simulink model "sltestCustomSourceSinkExample"  (R2016a)
settings: Solver=FixedStepDiscrete  SolverMode=SingleTasking  StartTime=0.0  StopTime=10  FixedStep=0.01  RelTol=1e-5  AbsTol=1e-6
model workspace (MAT data in the model file):
  PressEst = [0.806253176324 0.553142316929 0.37151500209 0.277667903103 0.220198954207 0.181288665766 0.153200000489 0.115431020872 0.0913067476324 0.0746519188607 0.0625231108324 0.0533383634277 ... (306 elements, 18x17)]
  PressVect = [0.05 0.1 0.15 0.2 0.25 0.3 0.35 0.4 0.45 0.5 0.55 0.6 0.65 0.7 0.75 0.8 0.85 0.9 0.95]
  PumpCon = [-0.0556348 -0.0022828 0.0256932 0.0435188 0.0562692 0.0661194857143 0.0741572 0.08697 0.0972452 0.106070342857 0.1139892 0.121303866667 ... (342 elements, 18x19)]
  RampRateKiX = [100 200 300 400 500 600]
  RampRateKiY = [0 0.2 0.4 0.6 0.8 1]
  RampRateKiZ = [0.012  0.024  0.036  0.048  0.06  0.072; 0.024  0.048  0.072  0.096  0.12  0.144; 0.036  0.072  0.108  0.144  0.18  0.216; 0.048  0.096  0.144  0.192  0.24  0.288; 0.06  0.12  0.18  0.24  0.3  0.36; 0.072  0.144  0.216  0.288  0.36  0.432]
  SpeedEst = [471.837839721 550.80940091 777.559313277 1080.9243499 1418.36795322 1769.7468768 2125.37309264 2480.20345067 2831.37796793 3177.14006959 3516.32917143 4064.90417867 ... (323 elements, 17x19)]
  SpeedVect = [50 75 100 125 150 175 200 250 300 350 400 450 500 600 700 800 900 1000]
  ThrotEst = [0 0 0 0 0 0 0 0 0 0 0 0 ... (342 elements, 18x19)]
  ThrotVect = [0 3 6 9 12 15 18 21 24 27 30 35 46 57 68 79 90]
  hys = 25
  max_ego = 1.2
  max_press = 0.95
  max_speed = 628
  max_throt = 90
  min_press = 0.05
  min_speed = 50
  min_throt = 3
  st_range = 0.0001
  zero_thresh = 250
Description:
  | This is a model of a fuel control system where Stateflow(R) is used to handle the fault management of the system.
  | The system contains four separate sensors: a throttle sensor, a speed sensor, an oxygen sensor, and a pressure sensor.
  | Each of these sensors is represented by a parallel state in Stateflow.  Each parallel state contains two substates, a
  | normal state and a failed state (the exception being the oxygen sensor, which also contains a warmup state).
  | 
  | If any of the sensor readings is outside an acceptable range, then a fault is registered in Stateflow, and the
  | substate of the corresponding subsystem transitions to the failed state.  If a subsystem recovers, it can
  | transition back to the normal state.  The number of failures in the system at any given time is represented
  | in the Fail parallel state.
  | 
  | The last parallel state in the Stateflow chart is called Fueling_Mode.  This state regulates the oxygen to
  | fuel mixture ratio.  If a failure is detected, then the oxygen to fuel ratio is increased.  If multiple failures
  | are detected, then the fuel system is disabled until there are no longer multiple failures in the system.
settings Model: ModifiedByFormat=The MathWorks Inc.  ExtModeTrigMode=oneshot  ExtModeArmWhenConnect=off  ExtModeAutoUpdateStatusClock=off  Creator=The MathWorks, Inc.  LastModifiedBy=The MathWorks Inc.
settings DataIOCC: SaveFormat=StructureWithTime  SaveOutput=off  SignalLogging=off  SaveTime=off  SignalLoggingName=dataout
settings OptimizationCC: DefaultParameterBehavior=Inlined  UseDivisionForNetSlopeComputation=UseDivisionForReciprocalsOfIntegersOnly  InlineInvariantSignals=on  EnhancedBackFolding=on  StrengthReduction=on  PassReuseOutputArgsThreshold=0  ExpressionDepthLimit=2147483647  EfficientFloat2IntCast=on
settings DebuggingCC: SignalInfNanChecking=error  SaveWithParameterizedLinksMsg=none  UnderspecifiedInitializationDetection=Classic  CheckExecutionContextPreStartOutputMsg=on  CheckExecutionContextRuntimeOutputMsg=on  IntegerOverflowMsg=none  ParameterDowncastMsg=warning  ParameterOverflowMsg=none  ParameterPrecisionLossMsg=none  UnderSpecifiedDataTypeMsg=warning  FcnCallInpInsideContextMsg=UseLocalSettings  UniqueDataStoreMsg=error  BusObjectLabelMismatch=error  StateNameClashWarn=warning  StrictBusMsg=ErrorOnBusTreatedAsVector  IntegerSaturationMsg=none
settings HardwareCC: ProdBitPerPointer=32  ProdLargestAtomicFloat=None  ProdWordSize=32  ProdHWDeviceType=Specified
settings ModelReferenceCC: PropagateSignalLabelsOutOfModel=off
settings SFSimCC: SimParseCustomCode=off
settings RTWCC: Description=Generic Real-Time Target  GenerateReport=on  RTWVerbose=off  LaunchReport=on
settings CodeAppCC: ForceParamTrailComments=on
settings ConfigComp: CovPath=/fuel_rate_control/control_logic  CovSFcnEnable=off

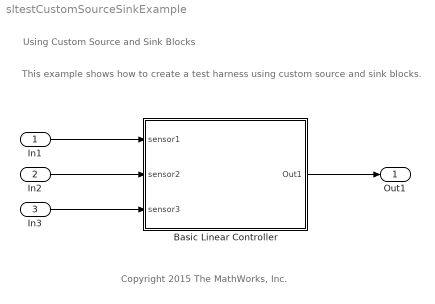
== system sltestCustomSourceSinkExample ==
  note: This example shows how to create a test harness using custom source and sink blocks.
  note: Using Custom Source and Sink Blocks
  note: Copyright 2015 The MathWorks, Inc.
  In1 : Inport  OutDataTypeStr=double  PortDimensions=1
  In2 : Inport  Port=2  OutDataTypeStr=double  PortDimensions=1
  In3 : Inport  Port=3  OutDataTypeStr=double  PortDimensions=1
  Basic Linear Controller : Subsystem  VariantControl=VSS_LINEAR_CONTROLLER
  Out1 : Outport
  wires:
  In2/1 -> Basic Linear Controller/2(sensor2)
  In1/1 -> Basic Linear Controller/1(sensor1)
  In3/1 -> Basic Linear Controller/3(sensor3)
  Basic Linear Controller/1(Out1) -> Out1/1

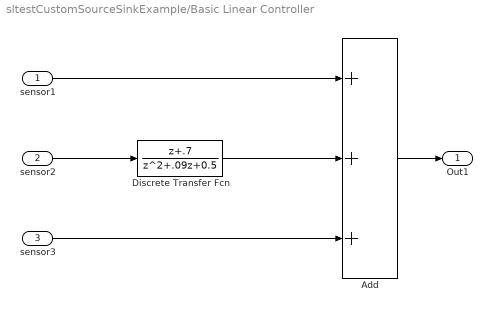
== system sltestCustomSourceSinkExample/Basic Linear Controller ==
  sensor1 : Inport
  sensor2 : Inport  Port=2
  sensor3 : Inport  Port=3
  Add : Sum  Inputs=+++
  Discrete Transfer Fcn : DiscreteTransferFcn  Numerator=[1 .7]  Denominator=[1 .09 0.5]  SampleTime=.01
  Out1 : Outport
  wires:
  sensor2/1 -> Discrete Transfer Fcn/1
  Discrete Transfer Fcn/1 -> Add/2
  sensor3/1 -> Add/3
  sensor1/1 -> Add/1
  Add/1 -> Out1/1
